simulink model "Bslope"  (R2022b)
settings: Solver=VariableStepAuto  StartTime=0.0  StopTime=70  FixedStep=0.01  MinStep=0.001  RelTol=1e-3  EnableMultiTasking=on
values from neighbouring files (symbols this model uses):
  Y = zeros(leg_num,1)    [Kimura.m]
undefined symbols (not defined in the file or in its folder): X, Z
libraries: sm_lib x84, nesl_utility x30, Contact_Forces_Lib x16, simulink_extras x12, robotcorelib x1
(part 3 of 3)

== system Bslope/Subsystem1/left_4 ==
  left_2 : sm_lib/Body Elements/File Solid  ExtGeomFileName=C:\Users\Administrator\Desktop\simulation\zuizhong\dog_1\left_2.stl  UnitType=Custom  ExtGeomFileUnits=mm  StepReaderType=HEX  ExportConvexHullGeometry=off  InertiaType=CalculateFromGeometry  Mass=1  MassUnits=kg  CenterOfMass=[0 0 0]  CenterOfMassUnits=m  MomentsOfInertia=[1 1 1]  MomentsOfInertiaUnits=kg*m^2  ProductsOfInertia=[0 0 0]  ProductsOfInertiaUnits=kg*m^2  BasedOnType=Density  Density=1000  DensityUnits=kg/m^3  DoExposeReferenceFrame=on  SerializedFrames=<Frames/>  GraphicType=FromGeometry  MarkerShape=Sphere  MarkerSize=10  GraphicVisPropType=SimpleVisualProperties  GraphicDiffuseColor=[0.5 0.5 0.5]  GraphicSpecularColor=[0.5 0.5 0.5 1.0]  GraphicAmbientColor=[0.15 0.15 0.15 1.0]  GraphicEmissiveColor=[0.0 0.0 0.0 1.0]  GraphicShininess=75  GraphicOpacity=1.0
  xyz2 : sm_lib/Frames and Transforms/Rigid Transform  TranslationMethod=Cartesian  TranslationStandardOffset=0  TranslationLengthUnit=mm  TranslationStandardAxis=+X  TranslationCartesianOffset=[-14.5 -107.5 0]  TranslationROffset=0  TranslationROffsetUnits=m  TranslationZOffset=0  TranslationZOffsetUnits=m  TranslationThetaOffset=0  TranslationThetaOffsetUnits=deg  RotationMethod=None  RotationAngleUnits=deg  RotationStandardAxis=+Y  RotationAngle=90  RotationArbitraryAxis=[0 0 1]  FollAlignAxisA=+X  BaseAlignAxisA=+Y  FollAlignAxisB=+Y  BaseAlignAxisB=+Z  RotationSequenceAxes=FollowerAxes  RotationSequence=XYX  RotationSequenceAngles=[0 0 0]  RotationSequenceAnglesUnits=deg  RotationMatrix=[1 0 0; 0 1 0; 0 0 1]  Quaternion=[1 0 0 0]
  Conn1 : PMIOPort  Side=Left
  Conn2 : PMIOPort  Port=2  Side=Right
  connections:
  Conn2/RConn1 -- xyz2/RConn1
  Conn1/RConn1 -- left_2/RConn1 -- xyz2/LConn1

== system Bslope/Subsystem1/letf_1 ==
  left_1 : sm_lib/Body Elements/File Solid  ExtGeomFileName=C:\Users\Administrator\Desktop\simulation\zuizhong\dog_1\left_3.stl  UnitType=Custom  ExtGeomFileUnits=mm  StepReaderType=HEX  ExportConvexHullGeometry=off  InertiaType=CalculateFromGeometry  Mass=1  MassUnits=kg  CenterOfMass=[0 0 0]  CenterOfMassUnits=m  MomentsOfInertia=[1 1 1]  MomentsOfInertiaUnits=kg*m^2  ProductsOfInertia=[0 0 0]  ProductsOfInertiaUnits=kg*m^2  BasedOnType=Density  Density=1000  DensityUnits=kg/m^3  DoExposeReferenceFrame=on  SerializedFrames=<Frames/>  GraphicType=FromGeometry  MarkerShape=Sphere  MarkerSize=10  GraphicVisPropType=SimpleVisualProperties  GraphicDiffuseColor=[0.5 0.5 0.5]  GraphicSpecularColor=[0.5 0.5 0.5 1.0]  GraphicAmbientColor=[0.15 0.15 0.15 1.0]  GraphicEmissiveColor=[0.0 0.0 0.0 1.0]  GraphicShininess=75  GraphicOpacity=1.0
  xyz1 : sm_lib/Frames and Transforms/Rigid Transform  TranslationMethod=None  TranslationStandardOffset=30  TranslationLengthUnit=mm  TranslationStandardAxis=+Z  TranslationCartesianOffset=[-14.5 -107.5 0]  TranslationROffset=0  TranslationROffsetUnits=m  TranslationZOffset=0  TranslationZOffsetUnits=m  TranslationThetaOffset=0  TranslationThetaOffsetUnits=deg  RotationMethod=StandardAxis  RotationAngleUnits=deg  RotationStandardAxis=+Z  RotationAngle=90  RotationArbitraryAxis=[0 0 1]  FollAlignAxisA=+X  BaseAlignAxisA=+Y  FollAlignAxisB=+Y  BaseAlignAxisB=+Z  RotationSequenceAxes=FollowerAxes  RotationSequence=XYX  RotationSequenceAngles=[0 0 0]  RotationSequenceAnglesUnits=deg  RotationMatrix=[1 0 0; 0 1 0; 0 0 1]  Quaternion=[1 0 0 0]
  xyz2 : sm_lib/Frames and Transforms/Rigid Transform  TranslationMethod=Cartesian  TranslationStandardOffset=30  TranslationLengthUnit=mm  TranslationStandardAxis=+Z  TranslationCartesianOffset=[122.5 -2.5 0]  TranslationROffset=0  TranslationROffsetUnits=m  TranslationZOffset=0  TranslationZOffsetUnits=m  TranslationThetaOffset=0  TranslationThetaOffsetUnits=deg  RotationMethod=None  RotationAngleUnits=deg  RotationStandardAxis=+Z  RotationAngle=-90  RotationArbitraryAxis=[0 0 1]  FollAlignAxisA=+X  BaseAlignAxisA=+Y  FollAlignAxisB=+Y  BaseAlignAxisB=+Z  RotationSequenceAxes=FollowerAxes  RotationSequence=XYX  RotationSequenceAngles=[0 0 0]  RotationSequenceAnglesUnits=deg  RotationMatrix=[1 0 0; 0 1 0; 0 0 1]  Quaternion=[1 0 0 0]
  xyz3 : sm_lib/Frames and Transforms/Rigid Transform  TranslationMethod=None  TranslationStandardOffset=30  TranslationLengthUnit=mm  TranslationStandardAxis=+Z  TranslationCartesianOffset=[-14.5 -107.5 0]  TranslationROffset=0  TranslationROffsetUnits=m  TranslationZOffset=0  TranslationZOffsetUnits=m  TranslationThetaOffset=0  TranslationThetaOffsetUnits=deg  RotationMethod=StandardAxis  RotationAngleUnits=deg  RotationStandardAxis=+X  RotationAngle=180  RotationArbitraryAxis=[0 0 1]  FollAlignAxisA=+X  BaseAlignAxisA=+Y  FollAlignAxisB=+Y  BaseAlignAxisB=+Z  RotationSequenceAxes=FollowerAxes  RotationSequence=XYX  RotationSequenceAngles=[0 0 0]  RotationSequenceAnglesUnits=deg  RotationMatrix=[1 0 0; 0 1 0; 0 0 1]  Quaternion=[1 0 0 0]
  xyz4 : sm_lib/Frames and Transforms/Rigid Transform  TranslationMethod=StandardAxis  TranslationStandardOffset=33  TranslationLengthUnit=mm  TranslationStandardAxis=+Z  TranslationCartesianOffset=[-14.5 -107.5 0]  TranslationROffset=0  TranslationROffsetUnits=m  TranslationZOffset=0  TranslationZOffsetUnits=m  TranslationThetaOffset=0  TranslationThetaOffsetUnits=deg  RotationMethod=None  RotationAngleUnits=deg  RotationStandardAxis=+X  RotationAngle=180  RotationArbitraryAxis=[0 0 1]  FollAlignAxisA=+X  BaseAlignAxisA=+Y  FollAlignAxisB=+Y  BaseAlignAxisB=+Z  RotationSequenceAxes=FollowerAxes  RotationSequence=XYX  RotationSequenceAngles=[0 0 0]  RotationSequenceAnglesUnits=deg  RotationMatrix=[1 0 0; 0 1 0; 0 0 1]  Quaternion=[1 0 0 0]
  Conn1 : PMIOPort  Side=Left
  Conn2 : PMIOPort  Port=2  Side=Right
  connections:
  Conn2/RConn1 -- xyz2/RConn1
  xyz3/LConn1 -- xyz4/RConn1
  xyz2/LConn1 -- left_1/RConn1 -- xyz1/RConn1
  xyz4/LConn1 -- Conn1/RConn1
  xyz1/LConn1 -- xyz3/RConn1

== system Bslope/Subsystem2/right_4 ==
  right_1 : sm_lib/Body Elements/File Solid  ExtGeomFileName=C:\Users\Administrator\Desktop\simulation\zuizhong\dog_1\right_1.stl  UnitType=Custom  ExtGeomFileUnits=mm  StepReaderType=HEX  ExportConvexHullGeometry=off  InertiaType=CalculateFromGeometry  Mass=1  MassUnits=kg  CenterOfMass=[0 0 0]  CenterOfMassUnits=m  MomentsOfInertia=[1 1 1]  MomentsOfInertiaUnits=kg*m^2  ProductsOfInertia=[0 0 0]  ProductsOfInertiaUnits=kg*m^2  BasedOnType=Density  Density=1000  DensityUnits=kg/m^3  DoExposeReferenceFrame=on  SerializedFrames=<Frames/>  GraphicType=FromGeometry  MarkerShape=Sphere  MarkerSize=10  GraphicVisPropType=SimpleVisualProperties  GraphicDiffuseColor=[0.5 0.5 0.5]  GraphicSpecularColor=[0.5 0.5 0.5 1.0]  GraphicAmbientColor=[0.15 0.15 0.15 1.0]  GraphicEmissiveColor=[0.0 0.0 0.0 1.0]  GraphicShininess=75  GraphicOpacity=1.0
  xyz1 : sm_lib/Frames and Transforms/Rigid Transform  TranslationMethod=StandardAxis  TranslationStandardOffset=5  TranslationLengthUnit=mm  TranslationStandardAxis=+Z  TranslationCartesianOffset=[0 0 40]  TranslationROffset=0  TranslationROffsetUnits=m  TranslationZOffset=0  TranslationZOffsetUnits=m  TranslationThetaOffset=0  TranslationThetaOffsetUnits=deg  RotationMethod=StandardAxis  RotationAngleUnits=deg  RotationStandardAxis=+X  RotationAngle=180  RotationArbitraryAxis=[0 0 1]  FollAlignAxisA=+X  BaseAlignAxisA=+Y  FollAlignAxisB=+Y  BaseAlignAxisB=+Z  RotationSequenceAxes=FollowerAxes  RotationSequence=XYX  RotationSequenceAngles=[0 0 0]  RotationSequenceAnglesUnits=deg  RotationMatrix=[1 0 0; 0 1 0; 0 0 1]  Quaternion=[1 0 0 0]
  xyz2 : sm_lib/Frames and Transforms/Rigid Transform  TranslationMethod=Cartesian  TranslationStandardOffset=0  TranslationLengthUnit=mm  TranslationStandardAxis=+X  TranslationCartesianOffset=[-27.5 0 -11.3]  TranslationROffset=0  TranslationROffsetUnits=m  TranslationZOffset=0  TranslationZOffsetUnits=m  TranslationThetaOffset=0  TranslationThetaOffsetUnits=deg  RotationMethod=StandardAxis  RotationAngleUnits=deg  RotationStandardAxis=+Y  RotationAngle=90  RotationArbitraryAxis=[0 0 1]  FollAlignAxisA=+X  BaseAlignAxisA=+Y  FollAlignAxisB=+Y  BaseAlignAxisB=+Z  RotationSequenceAxes=FollowerAxes  RotationSequence=XYX  RotationSequenceAngles=[0 0 0]  RotationSequenceAnglesUnits=deg  RotationMatrix=[1 0 0; 0 1 0; 0 0 1]  Quaternion=[1 0 0 0]
  Conn1 : PMIOPort  Side=Left
  Conn2 : PMIOPort  Port=2  Side=Right
  connections:
  Conn2/RConn1 -- xyz2/RConn1
  xyz2/LConn1 -- right_1/RConn1 -- xyz1/LConn1
  xyz1/RConn1 -- Conn1/RConn1

== system Bslope/Subsystem2/right_5 ==
  right_2 : sm_lib/Body Elements/File Solid  ExtGeomFileName=C:\Users\Administrator\Desktop\simulation\zuizhong\dog_1\right_2.stl  UnitType=Custom  ExtGeomFileUnits=mm  StepReaderType=HEX  ExportConvexHullGeometry=off  InertiaType=CalculateFromGeometry  Mass=1  MassUnits=kg  CenterOfMass=[0 0 0]  CenterOfMassUnits=m  MomentsOfInertia=[1 1 1]  MomentsOfInertiaUnits=kg*m^2  ProductsOfInertia=[0 0 0]  ProductsOfInertiaUnits=kg*m^2  BasedOnType=Density  Density=1000  DensityUnits=kg/m^3  DoExposeReferenceFrame=on  SerializedFrames=<Frames/>  GraphicType=FromGeometry  MarkerShape=Sphere  MarkerSize=10  GraphicVisPropType=SimpleVisualProperties  GraphicDiffuseColor=[0.5 0.5 0.5]  GraphicSpecularColor=[0.5 0.5 0.5 1.0]  GraphicAmbientColor=[0.15 0.15 0.15 1.0]  GraphicEmissiveColor=[0.0 0.0 0.0 1.0]  GraphicShininess=75  GraphicOpacity=1.0
  xyz1 : sm_lib/Frames and Transforms/Rigid Transform  TranslationMethod=Cartesian  TranslationStandardOffset=0  TranslationLengthUnit=mm  TranslationStandardAxis=+X  TranslationCartesianOffset=[-14.5 -107.5 0]  TranslationROffset=0  TranslationROffsetUnits=m  TranslationZOffset=0  TranslationZOffsetUnits=m  TranslationThetaOffset=0  TranslationThetaOffsetUnits=deg  RotationMethod=None  RotationAngleUnits=deg  RotationStandardAxis=+Y  RotationAngle=90  RotationArbitraryAxis=[0 0 1]  FollAlignAxisA=+X  BaseAlignAxisA=+Y  FollAlignAxisB=+Y  BaseAlignAxisB=+Z  RotationSequenceAxes=FollowerAxes  RotationSequence=XYX  RotationSequenceAngles=[0 0 0]  RotationSequenceAnglesUnits=deg  RotationMatrix=[1 0 0; 0 1 0; 0 0 1]  Quaternion=[1 0 0 0]
  Conn1 : PMIOPort  Side=Left
  Conn2 : PMIOPort  Port=2  Side=Right
  connections:
  Conn2/RConn1 -- xyz1/RConn1
  Conn1/RConn1 -- right_2/RConn1 -- xyz1/LConn1

== system Bslope/Subsystem2/right_6 ==
  right_3 : sm_lib/Body Elements/File Solid  ExtGeomFileName=C:\Users\Administrator\Desktop\simulation\zuizhong\dog_1\right_3.stl  UnitType=Custom  ExtGeomFileUnits=mm  StepReaderType=HEX  ExportConvexHullGeometry=off  InertiaType=CalculateFromGeometry  Mass=1  MassUnits=kg  CenterOfMass=[0 0 0]  CenterOfMassUnits=m  MomentsOfInertia=[1 1 1]  MomentsOfInertiaUnits=kg*m^2  ProductsOfInertia=[0 0 0]  ProductsOfInertiaUnits=kg*m^2  BasedOnType=Density  Density=1000  DensityUnits=kg/m^3  DoExposeReferenceFrame=on  SerializedFrames=<Frames/>  GraphicType=FromGeometry  MarkerShape=Sphere  MarkerSize=10  GraphicVisPropType=SimpleVisualProperties  GraphicDiffuseColor=[0.5 0.5 0.5]  GraphicSpecularColor=[0.5 0.5 0.5 1.0]  GraphicAmbientColor=[0.15 0.15 0.15 1.0]  GraphicEmissiveColor=[0.0 0.0 0.0 1.0]  GraphicShininess=75  GraphicOpacity=1.0
  xyz1 : sm_lib/Frames and Transforms/Rigid Transform  TranslationMethod=None  TranslationStandardOffset=30  TranslationLengthUnit=mm  TranslationStandardAxis=+Z  TranslationCartesianOffset=[-14.5 -107.5 0]  TranslationROffset=0  TranslationROffsetUnits=m  TranslationZOffset=0  TranslationZOffsetUnits=m  TranslationThetaOffset=0  TranslationThetaOffsetUnits=deg  RotationMethod=StandardAxis  RotationAngleUnits=deg  RotationStandardAxis=+X  RotationAngle=180  RotationArbitraryAxis=[0 0 1]  FollAlignAxisA=+X  BaseAlignAxisA=+Y  FollAlignAxisB=+Y  BaseAlignAxisB=+Z  RotationSequenceAxes=FollowerAxes  RotationSequence=XYX  RotationSequenceAngles=[0 0 0]  RotationSequenceAnglesUnits=deg  RotationMatrix=[1 0 0; 0 1 0; 0 0 1]  Quaternion=[1 0 0 0]
  xyz2 : sm_lib/Frames and Transforms/Rigid Transform  TranslationMethod=Cartesian  TranslationStandardOffset=30  TranslationLengthUnit=mm  TranslationStandardAxis=+Z  TranslationCartesianOffset=[122.5 -2.5 0]  TranslationROffset=0  TranslationROffsetUnits=m  TranslationZOffset=0  TranslationZOffsetUnits=m  TranslationThetaOffset=0  TranslationThetaOffsetUnits=deg  RotationMethod=None  RotationAngleUnits=deg  RotationStandardAxis=+Z  RotationAngle=-90  RotationArbitraryAxis=[0 0 1]  FollAlignAxisA=+X  BaseAlignAxisA=+Y  FollAlignAxisB=+Y  BaseAlignAxisB=+Z  RotationSequenceAxes=FollowerAxes  RotationSequence=XYX  RotationSequenceAngles=[0 0 0]  RotationSequenceAnglesUnits=deg  RotationMatrix=[1 0 0; 0 1 0; 0 0 1]  Quaternion=[1 0 0 0]
  xyz3 : sm_lib/Frames and Transforms/Rigid Transform  TranslationMethod=None  TranslationStandardOffset=-5  TranslationLengthUnit=mm  TranslationStandardAxis=+Z  TranslationCartesianOffset=[-14.5 -107.5 0]  TranslationROffset=0  TranslationROffsetUnits=m  TranslationZOffset=0  TranslationZOffsetUnits=m  TranslationThetaOffset=0  TranslationThetaOffsetUnits=deg  RotationMethod=StandardAxis  RotationAngleUnits=deg  RotationStandardAxis=+Z  RotationAngle=90  RotationArbitraryAxis=[0 0 1]  FollAlignAxisA=+X  BaseAlignAxisA=+Y  FollAlignAxisB=+Y  BaseAlignAxisB=+Z  RotationSequenceAxes=FollowerAxes  RotationSequence=XYX  RotationSequenceAngles=[0 0 0]  RotationSequenceAnglesUnits=deg  RotationMatrix=[1 0 0; 0 1 0; 0 0 1]  Quaternion=[1 0 0 0]
  xyz4 : sm_lib/Frames and Transforms/Rigid Transform  TranslationMethod=StandardAxis  TranslationStandardOffset=-33  TranslationLengthUnit=mm  TranslationStandardAxis=+Z  TranslationCartesianOffset=[-14.5 -107.5 0]  TranslationROffset=0  TranslationROffsetUnits=m  TranslationZOffset=0  TranslationZOffsetUnits=m  TranslationThetaOffset=0  TranslationThetaOffsetUnits=deg  RotationMethod=None  RotationAngleUnits=deg  RotationStandardAxis=+X  RotationAngle=180  RotationArbitraryAxis=[0 0 1]  FollAlignAxisA=+X  BaseAlignAxisA=+Y  FollAlignAxisB=+Y  BaseAlignAxisB=+Z  RotationSequenceAxes=FollowerAxes  RotationSequence=XYX  RotationSequenceAngles=[0 0 0]  RotationSequenceAnglesUnits=deg  RotationMatrix=[1 0 0; 0 1 0; 0 0 1]  Quaternion=[1 0 0 0]
  Conn1 : PMIOPort  Side=Left
  Conn2 : PMIOPort  Port=2  Side=Right
  connections:
  xyz1/LConn1 -- xyz4/RConn1
  right_3/RConn1 -- xyz2/LConn1 -- xyz3/RConn1
  Conn2/RConn1 -- xyz2/RConn1
  xyz4/LConn1 -- Conn1/RConn1
  xyz3/LConn1 -- xyz1/RConn1

== system Bslope/步态规划1/Subsystem ==
  Clock : simulink_extras/Flip Flops/Clock  period=1
  Clock1 : simulink_extras/Flip Flops/Clock  period=0.5
  Integrator1 : Integrator
  MATLAB Function : MATLAB Function  TreatAsAtomicUnit=on
  MATLAB Function1 : MATLAB Function  TreatAsAtomicUnit=on
  Product : Product
  Out1 : Outport  VectorParamsAs1DForOutWhenUnconnected=off
  wires:
  Product/1 -> Out1/1
  Integrator1/1 -> Product/1
  Clock/1 -> MATLAB Function/1(u)
  MATLAB Function/1(y) -> Product/2
  Clock1/1 -> MATLAB Function1/1(u)
  MATLAB Function1/1(y) -> Integrator1/1

== system Bslope/步态规划1/Subsystem1 ==
  Clock : simulink_extras/Flip Flops/Clock  period=2
  Clock1 : simulink_extras/Flip Flops/Clock  period=1
  Integrator1 : Integrator
  MATLAB Function : MATLAB Function  TreatAsAtomicUnit=on
  MATLAB Function1 : MATLAB Function  TreatAsAtomicUnit=on
  Product : Product
  Out1 : Outport  VectorParamsAs1DForOutWhenUnconnected=off
  wires:
  Product/1 -> Out1/1
  Integrator1/1 -> Product/1
  Clock/1 -> MATLAB Function/1(u)
  MATLAB Function/1(y) -> Product/2
  Clock1/1 -> MATLAB Function1/1(u)
  MATLAB Function1/1(y) -> Integrator1/1

== system Bslope/步态规划2/Subsystem ==
  Clock : simulink_extras/Flip Flops/Clock  period=1
  Clock1 : simulink_extras/Flip Flops/Clock  period=0.5
  Integrator1 : Integrator
  MATLAB Function : MATLAB Function  TreatAsAtomicUnit=on
  MATLAB Function1 : MATLAB Function  TreatAsAtomicUnit=on
  Product : Product
  Out1 : Outport  VectorParamsAs1DForOutWhenUnconnected=off
  wires:
  Product/1 -> Out1/1
  Integrator1/1 -> Product/1
  Clock/1 -> MATLAB Function/1(u)
  MATLAB Function/1(y) -> Product/2
  Clock1/1 -> MATLAB Function1/1(u)
  MATLAB Function1/1(y) -> Integrator1/1

== system Bslope/步态规划2/Subsystem1 ==
  Clock : simulink_extras/Flip Flops/Clock  period=2
  Clock1 : simulink_extras/Flip Flops/Clock  period=1
  Integrator1 : Integrator
  MATLAB Function : MATLAB Function  TreatAsAtomicUnit=on
  MATLAB Function1 : MATLAB Function  TreatAsAtomicUnit=on
  Product : Product
  Out1 : Outport  VectorParamsAs1DForOutWhenUnconnected=off
  wires:
  Product/1 -> Out1/1
  Integrator1/1 -> Product/1
  Clock/1 -> MATLAB Function/1(u)
  MATLAB Function/1(y) -> Product/2
  Clock1/1 -> MATLAB Function1/1(u)
  MATLAB Function1/1(y) -> Integrator1/1

== system Bslope/步态规划3/Subsystem ==
  Clock : simulink_extras/Flip Flops/Clock  period=4
  Clock1 : simulink_extras/Flip Flops/Clock  period=2
  Integrator1 : Integrator
  MATLAB Function : MATLAB Function  TreatAsAtomicUnit=on
  MATLAB Function1 : MATLAB Function  TreatAsAtomicUnit=on
  Product : Product
  Out1 : Outport  VectorParamsAs1DForOutWhenUnconnected=off
  wires:
  Product/1 -> Out1/1
  Integrator1/1 -> Product/1
  Clock/1 -> MATLAB Function/1(u)
  MATLAB Function/1(y) -> Product/2
  Clock1/1 -> MATLAB Function1/1(u)
  MATLAB Function1/1(y) -> Integrator1/1

== system Bslope/步态规划3/Subsystem1 ==
  Clock : simulink_extras/Flip Flops/Clock  period=8
  Clock1 : simulink_extras/Flip Flops/Clock  period=4
  Integrator1 : Integrator
  MATLAB Function : MATLAB Function  TreatAsAtomicUnit=on
  MATLAB Function1 : MATLAB Function  TreatAsAtomicUnit=on
  Product : Product
  Out1 : Outport  VectorParamsAs1DForOutWhenUnconnected=off
  wires:
  Product/1 -> Out1/1
  Integrator1/1 -> Product/1
  Clock/1 -> MATLAB Function/1(u)
  MATLAB Function/1(y) -> Product/2
  Clock1/1 -> MATLAB Function1/1(u)
  MATLAB Function1/1(y) -> Integrator1/1

== matlab function Bslope/步态规划1/Subsystem/MATLAB Function ==
  data: u input; y output
function y = fcn(u)
if u==0
    y = -1;
else
    y=1;
end
end

== matlab function Bslope/步态规划1/Subsystem/MATLAB Function1 ==
  data: u input; y output
function y = fcn(u)
if u==0
    y = -1;
else
    y=1;
end
end

== matlab function Bslope/步态规划1/Subsystem1/MATLAB Function ==
  data: u input; y output
function y = fcn(u)
if u==0
    y = -1;
else
    y=1;
end
end

== matlab function Bslope/步态规划1/Subsystem1/MATLAB Function1 ==
  data: u input; y output
function y = fcn(u)
if u==0
    y = -1;
else
    y=1;
end
end

== matlab function Bslope/步态规划2/0-Tm_x1 ==
  data: u input; x output; Tm input; S input
function x = fcn(u,Tm,S)


if u>0
   
    x =S*(u/Tm-1/(2*pi)*sin(2*pi*u/Tm));
else 
    u=-u;
    x =S*(u/Tm-1/(2*pi)*sin(2*pi*u/Tm));
end

== matlab function Bslope/步态规划2/0-Tm_x2 ==
  data: u input; x output; Tm input; S input
function x = fcn(u,Tm,S)

if u>0
    x =S*(u/Tm-1/(2*pi)*sin(2*pi*u/Tm));
else 
    u=-u;
     x =S*(u/Tm-1/(2*pi)*sin(2*pi*u/Tm));
end

== matlab function Bslope/步态规划2/0-Tm_y1 ==
  data: u input; y output; S input; Tm input; H input
function y = fcn(u,S,Tm,H)

n=4;
if u>0
    y=2*H*(u/Tm-1/(n*pi)*sin(n*pi*u/Tm)).*(u>=0&u<Tm/2)+2*H*(1-u/Tm+1/(n*pi)*sin(n*pi*u/Tm)).*(u>=Tm/2&u<Tm);;
else 
    y=0;
end

== matlab function Bslope/步态规划2/0-Tm_y2 ==
  data: u input; y output; S input; Tm input; H input
function y = fcn(u,S,Tm,H)

n=4;
if u>0
    y=2*H*(u/Tm-1/(n*pi)*sin(n*pi*u/Tm)).*(u>=0&u<Tm/2)+2*H*(1-u/Tm+1/(n*pi)*sin(n*pi*u/Tm)).*(u>=Tm/2&u<Tm);;
else 
    y=0;
end

== matlab function Bslope/步态规划2/Subsystem/MATLAB Function ==
  data: u input; y output
function y = fcn(u)
if u==0
    y = -1;
else
    y=1;
end
end

== matlab function Bslope/步态规划2/Subsystem/MATLAB Function1 ==
  data: u input; y output
function y = fcn(u)
if u==0
    y = -1;
else
    y=1;
end
end

== matlab function Bslope/步态规划2/Subsystem1/MATLAB Function ==
  data: u input; y output
function y = fcn(u)
if u==0
    y = -1;
else
    y=1;
end
end

== matlab function Bslope/步态规划2/Subsystem1/MATLAB Function1 ==
  data: u input; y output
function y = fcn(u)
if u==0
    y = -1;
else
    y=1;
end
end

== matlab function Bslope/逆运动学解算/MATLAB FR ==
  data: x input; alfa output; y input; z input; beta output; gamma output
function [alfa,beta,gamma]=xyztoang(x,y,z)
h=49.0;
hu=125.5899;
hl=116.0+20;

dyz=sqrt(y.^2+z.^2);
lyz=sqrt(dyz.^2-h.^2);
gamma_yz=-atan(y./z);
gamma_h_offset=-atan(h./lyz);
gamma=gamma_yz-gamma_h_offset;

lxzp=sqrt(lyz.^2+x.^2);
n=(lxzp.^2-hl^2-hu.^2)/(2*hu);
beta=-acos(n/hl);

alfa_xzp=-atan(x/lyz);
alfa_off=acos((hu+n)/lxzp);
alfa=(alfa_xzp+alfa_off);
end

== matlab function Bslope/步态规划3/0-Tm_x1 ==
  data: u input; x output; Tm input; S input
function x = fcn(u,Tm,S)


if u>0
   
    x =S*(u/Tm-1/(2*pi)*sin(2*pi*u/Tm));
else 
    u=-u;
    x =S*(u/Tm-1/(2*pi)*sin(2*pi*u/Tm));
end

== matlab function Bslope/步态规划3/0-Tm_x2 ==
  data: u input; x output; Tm input; S input
function x = fcn(u,Tm,S)

if u>0
    x =S*(u/Tm-1/(2*pi)*sin(2*pi*u/Tm));
else 
    u=-u;
     x =S*(u/Tm-1/(2*pi)*sin(2*pi*u/Tm));
end

== matlab function Bslope/步态规划3/0-Tm_y1 ==
  data: u input; y output; S input; Tm input; H input
function y = fcn(u,S,Tm,H)

n=4;
if u>0
    y=2*H*(u/Tm-1/(n*pi)*sin(n*pi*u/Tm)).*(u>=0&u<Tm/2)+2*H*(1-u/Tm+1/(n*pi)*sin(n*pi*u/Tm)).*(u>=Tm/2&u<Tm);;
else 
    y=0;
end

== matlab function Bslope/步态规划3/0-Tm_y2 ==
  data: u input; y output; S input; Tm input; H input
function y = fcn(u,S,Tm,H)

n=4;
if u>0
    y=2*H*(u/Tm-1/(n*pi)*sin(n*pi*u/Tm)).*(u>=0&u<Tm/2)+2*H*(1-u/Tm+1/(n*pi)*sin(n*pi*u/Tm)).*(u>=Tm/2&u<Tm);;
else 
    y=0;
end

== matlab function Bslope/步态规划3/Subsystem/MATLAB Function ==
  data: u input; y output
function y = fcn(u)
if u==0
    y = -1;
else
    y=1;
end
end

== matlab function Bslope/步态规划3/Subsystem/MATLAB Function1 ==
  data: u input; y output
function y = fcn(u)
if u==0
    y = -1;
else
    y=1;
end
end

== matlab function Bslope/步态规划3/Subsystem1/MATLAB Function ==
  data: u input; y output
function y = fcn(u)
if u==0
    y = -1;
else
    y=1;
end
end

== matlab function Bslope/步态规划3/Subsystem1/MATLAB Function1 ==
  data: u input; y output
function y = fcn(u)
if u==0
    y = -1;
else
    y=1;
end
end

== matlab function Bslope/逆运动学解算/ FL ==
  data: x input; alfa output; y input; z input; beta output; gamma output
function [alfa,beta,gamma]=xyztoang(x,y,z)
h=49.0;
hu=125.5899;
hl=116.0+20;

dyz=sqrt(y.^2+z.^2);
lyz=sqrt(dyz.^2-h.^2);
gamma_yz=-atan(y./z);
gamma_h_offset=-atan(h./lyz);
gamma=gamma_yz-gamma_h_offset;

lxzp=sqrt(lyz.^2+x.^2);
n=(lxzp.^2-hl^2-hu.^2)/(2*hu);
beta=-acos(n/hl);

alfa_xzp=-atan(x/lyz);
alfa_off=acos((hu+n)/lxzp);
alfa=(alfa_xzp+alfa_off);
end

== matlab function Bslope/逆运动学解算/MATLAB BL ==
  data: x input; alfa output; y input; z input; beta output; gamma output
function [alfa,beta,gamma]=xyztoang(x,y,z)
h=49.0;
hu=125.5899;
hl=116.0+20;

dyz=sqrt(y.^2+z.^2);
lyz=sqrt(dyz.^2-h.^2);
gamma_yz=-atan(y./z);
gamma_h_offset=-atan(h./lyz);
gamma=gamma_yz-gamma_h_offset;

lxzp=sqrt(lyz.^2+x.^2);
n=(lxzp.^2-hl^2-hu.^2)/(2*hu);
beta=-acos(n/hl);

alfa_xzp=-atan(x/lyz);
alfa_off=acos((hu+n)/lxzp);
alfa=(alfa_xzp+alfa_off);
end

== matlab function Bslope/逆运动学解算/MATLAB BR ==
  data: x input; alfa output; y input; z input; beta output; gamma output
function [alfa,beta,gamma]=xyztoang(x,y,z)
h=49.0;
hu=125.5899;
hl=116.0+20;

dyz=sqrt(y.^2+z.^2);
lyz=sqrt(dyz.^2-h.^2);
gamma_yz=-atan(y./z);
gamma_h_offset=-atan(h./lyz);
gamma=gamma_yz-gamma_h_offset;

lxzp=sqrt(lyz.^2+x.^2);
n=(lxzp.^2-hl^2-hu.^2)/(2*hu);
beta=-acos(n/hl);

alfa_xzp=-atan(x/lyz);
alfa_off=acos((hu+n)/lxzp);
alfa=(alfa_xzp+alfa_off);
end

== matlab function Bslope/步态规划1/0-Tm_x1 ==
  data: u input; x output; Tm input; S input
function x = fcn(u,Tm,S)


if u>0
   
    x =S*(u/Tm-1/(2*pi)*sin(2*pi*u/Tm));
else 
    u=-u;
    x =S*(u/Tm-1/(2*pi)*sin(2*pi*u/Tm));
end

== matlab function Bslope/步态规划1/0-Tm_x2 ==
  data: u input; x output; Tm input; S input
function x = fcn(u,Tm,S)

if u>0
    x =S*(u/Tm-1/(2*pi)*sin(2*pi*u/Tm));
else 
    u=-u;
     x =S*(u/Tm-1/(2*pi)*sin(2*pi*u/Tm));
end

== matlab function Bslope/步态规划1/0-Tm_y1 ==
  data: u input; y output; S input; Tm input; H input
function y = fcn(u,S,Tm,H)

n=4;
if u>0
    y=2*H*(u/Tm-1/(n*pi)*sin(n*pi*u/Tm)).*(u>=0&u<Tm/2)+2*H*(1-u/Tm+1/(n*pi)*sin(n*pi*u/Tm)).*(u>=Tm/2&u<Tm);;
else 
    y=0;
end

== matlab function Bslope/步态规划1/0-Tm_y2 ==
  data: u input; y output; S input; Tm input; H input
function y = fcn(u,S,Tm,H)

n=4;
if u>0
    y=2*H*(u/Tm-1/(n*pi)*sin(n*pi*u/Tm)).*(u>=0&u<Tm/2)+2*H*(1-u/Tm+1/(n*pi)*sin(n*pi*u/Tm)).*(u>=Tm/2&u<Tm);;
else 
    y=0;
end
